simulink library "DQ_SR_LIB_SIM"  (R2019b)
settings: Solver=VariableStepAuto  StartTime=0.0  StopTime=10.0  RelTol=1e-3  EnableMultiTasking=on
undefined symbols (not defined in the file): crossqm, II, II0, magnitude, SATFUNCNAME, X0, XCG0, xi0
(part 2 of 2)

== matlab function DQ_SR_LIB_SIM/DQ Kinematics fixed mass multiple systems/MATLAB Function2 ==
  data: t input; dy output; DCG output; state input size=[n_var,1]; CG input; II parameter; ext_f input size=[n_ext]; sys_gen_fun_NAME parameter; gravity_fun_NAME parameter; coll_v_ref data_store_memory; CONTACTABLE data_store_memory
function [dy,DCG] = DQ_coreMCM(t,state,CG,II,ext_f,sys_gen_fun_NAME,gravity_fun_NAME)
%#codegen


% cg variables
vcg=CG(1:3,:);
xcg=CG(4:6,:);


% user defined functions
sys_gen_fun=str2func(char(sys_gen_fun_NAME));
gravity_fun=str2func(char(gravity_fun_NAME));


% global coll_v_ref

% coll_v_ref

% system computation
[dy,DCG]=dynamicsMCM(t,state,xcg,vcg,II,ext_f,sys_gen_fun,gravity_fun);

== matlab function DQ_SR_LIB_SIM/DQ Kinematics fixed mass multiple systems/MATLAB Function3 ==
  data: t input; state input size=[n_var,1]; a output; CG input; II parameter; n_ext parameter; sys_gen_fun_NAME parameter; n_bodies parameter size=1; da output; coll_v_ref data_store_memory
function [a,da] = get_the_dq_state(t,state,CG,II,n_ext,sys_gen_fun_NAME,n_bodies)
%#codegen


% cg variables
vcg=CG(1:3,:);
xcg=CG(4:6,:);

% state dimension
n_var=length(state)/2;

% get state and its derivative
dx=state(1:n_var);
x=state(n_var+1:end);




% user defined functions
sys_gen_fun=str2func(char(sys_gen_fun_NAME));


% global coll_v_ref


% extract all the states
[SYSTEMS]=sys_gen_fun(x,dx,xcg,vcg,t,II,zeros(n_ext,1),[],[]);

% initialize
index=1;
[a,da]=deal(zeros(8,n_bodies));

for i=1:length(SYSTEMS)
    
    % get current system
    SYS=SYSTEMS(i);
    
    % enforce the constraints
    SYS=enforce_cg_constr(SYS);
    
    % % extract the state
    [a(:,index:(index+SYS.n_bodies-1)),da(:,index:(index+SYS.n_bodies-1))]=getfullstate(SYS,SYS.n_bodies);
    
    % adjourne index
    index=(index+SYS.n_bodies);
    
end




end

== matlab function DQ_SR_LIB_SIM/Utilities/Dq matrix/MATLAB Function ==
  data: u input; y output; fun_NAME parameter
function y = fcn(u,fun_NAME)
%#codegen

fun=str2func(char(fun_NAME));

y = fun(u);

== matlab function DQ_SR_LIB_SIM/Utilities/q matrix/MATLAB Function ==
  data: u input; y output; fun_NAME parameter
function y = fcn(u,fun_NAME)
%#codegen

fun=str2func(char(fun_NAME));

y = fun(u);

== matlab function DQ_SR_LIB_SIM/Utilities/Body velocity/MATLAB Function ==
  data: a input; d output; da input
function d = fcn(a,da)
%#codegen


QPT=crossqp(a(1:4))';
QPT=QPT(1:3,:);
dQPT=crossqp(da(1:4))';
dQPT=dQPT(1:3,:);


d=2*(QPT*da(5:8)+dQPT*a(5:8));

== matlab function DQ_SR_LIB_SIM/Utilities/Inertial velocity/MATLAB Function ==
  data: a input; d output; da input
function d = fcn(a,da)
%#codegen


QMT=crossqm(a(1:4))';
QMT=QMT(1:3,:);
dQMT=crossqm(da(1:4))';
dQMT=dQMT(1:3,:);

d=2*(QMT*da(5:8)+dQMT*a(5:8));

== matlab function DQ_SR_LIB_SIM/Utilities/q transform/MATLAB Function ==
  data: u input; y output; fun_NAME parameter
function y = fcn(u,fun_NAME)
%#codegen

fun=str2func(char(fun_NAME));

y = fun(u);

== matlab function DQ_SR_LIB_SIM/Utilities/quaternion product/MATLAB Function ==
  data: u input; y output; fun_NAME parameter; ISTRANSPOSE parameter
function y = fcn(u,fun_NAME,ISTRANSPOSE)
%#codegen

% extract function
fun=str2func(char(fun_NAME));
% evaluate function
y = fun(u);

if ISTRANSPOSE
   % traspose if required 
    y = y';
end

== matlab function DQ_SR_LIB_SIM/Utilities/dual quaternion product/MATLAB Function ==
  data: u input; y output; fun_NAME parameter; ISTRANSPOSE parameter
function y = fcn(u,fun_NAME,ISTRANSPOSE)
%#codegen

% extract function
fun=str2func(char(fun_NAME));
% evaluate function
y = fun(u);

if ISTRANSPOSE
   % traspose if required 
    y = y';
end

== matlab function DQ_SR_LIB_SIM/Utilities/Inertial dq/MATLAB Function ==
  data: a output; d input; q input
function a = fcn(d,q)
%#codegen


QM=crossqm(q);
QM=QM(:,1:3);

t = QM*d/2;

a = [q;t];

== matlab function DQ_SR_LIB_SIM/Utilities/dq normalizer/MATLAB Function ==
  data: u input; y output
function y = fcn(u)
%#codegen

% input
q = u(1:4);
t = u(5:8);

% normalize attitude quaternion
q = q/norm(q);

% normalize position quaternion
d = 2*crossqm(q)'*t;
t = .5*crossqm(q)*[d(1:3);0];

%output
y = [q;t];

== matlab function DQ_SR_LIB_SIM/Utilities/Dual quaternion selection/MATLAB Function ==
  data: a input; x parameter; y parameter; a_xy output
function a_xy = selectindex(a,x,y)
%#codegen
% select as output the index of elements and body

[~,n]=size(a);

if n==1
    % avoid null selection
    y=1;
end

% a_xy=zeros(8,8);

a_xy = a(x,y);
